simulink model "Sistema_Complejo"  (R2017b)
settings: Solver=FixedStepAuto  StartTime=0.0  StopTime=10.0  FixedStep=0.001  RelTol=1e-3
values from neighbouring files (symbols this model uses):
  B = 20    [Sistema_Complejo.m]    (also in Sistema_Sencillo.m)
  F = 100    [Sistema_Complejo.m]    (also in Sistema_Sencillo.m)
  K1 = 491.1    [Sistema_Complejo.m]
  K2 = 50    [Sistema_Complejo.m]
  K3 = 400    [Sistema_Complejo.m]
  M1 = 5.23    [Sistema_Complejo.m]
  M2 = 2.615    [Sistema_Complejo.m]
  ST = 1    [Sistema_Complejo.m]    (also in Sistema_Sencillo.m)
  VI = 0    [Sistema_Complejo.m]    (also in Sistema_Sencillo.m)
settings Model: Creator=DELL  LastModifiedBy=Wilmer
settings SFSimCC: SimUseLocalCustomCode=on
settings RTWCC: RTWUseLocalCustomCode=on
settings CodeAppCC: StateflowObjectComments=on

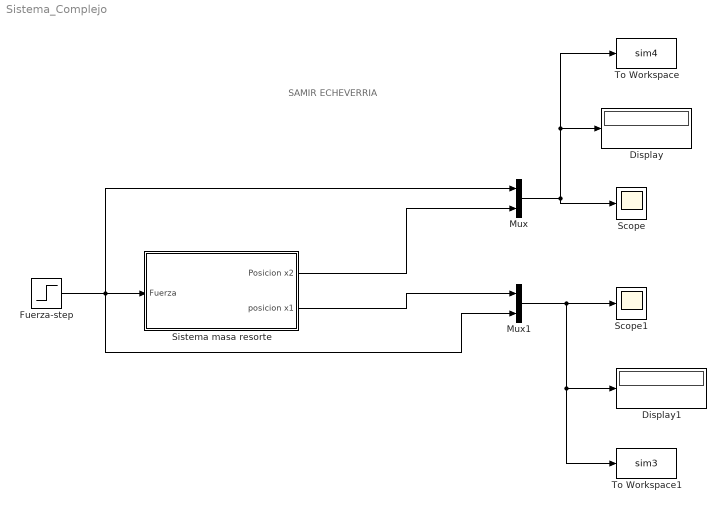
== system Sistema_Complejo ==
  note: SAMIR ECHEVERRIA
  Display : Display
  Display1 : Display
  Fuerza-step : Step  Time=ST  Before=VI  After=F  SampleTime=0
  Mux : Mux  Inputs=2
  Mux1 : Mux  Inputs=2
  Scope : Scope
  Scope1 : Scope
  Sistema masa resorte : Subsystem
  To Workspace : ToWorkspace  VariableName=sim4  SampleTime=-1
  To Workspace1 : ToWorkspace  VariableName=sim3  SampleTime=-1
  wires:
  Fuerza-step/1 -> Mux1/2, Mux/1, Sistema masa resorte/1(Fuerza)
  Sistema masa resorte/1(Posicion x2) -> Mux/2
  Mux/1 -> To Workspace/1, Display/1, Scope/1
  Sistema masa resorte/2("posicion x1 ") -> Mux1/1
  Mux1/1 -> To Workspace1/1, Display1/1, Scope1/1

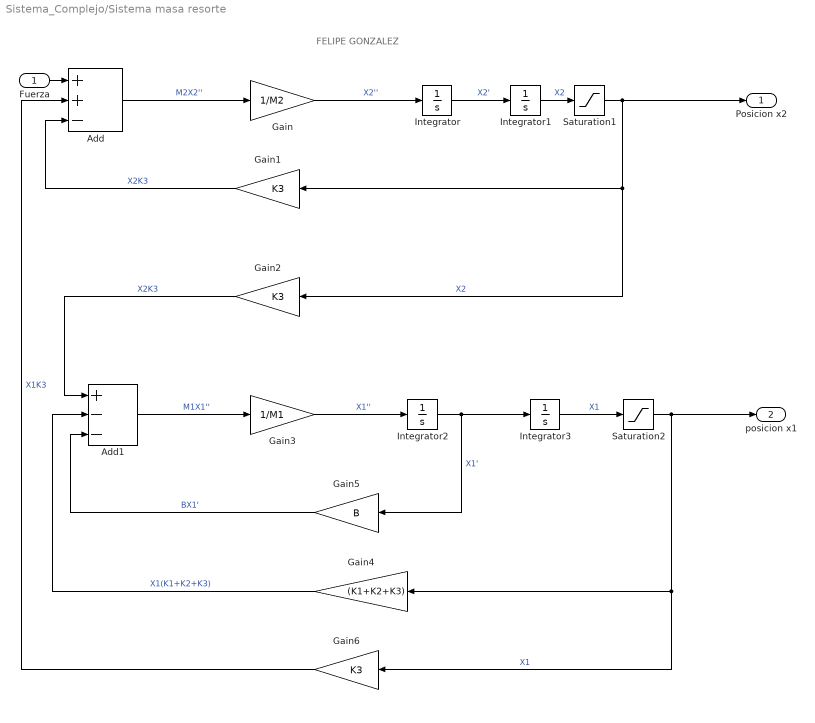
== system Sistema_Complejo/Sistema masa resorte ==
  note: FELIPE GONZALEZ
  Fuerza : Inport
  Add : Sum  Inputs=++-
  Add1 : Sum  Inputs=+--
  Gain : Gain  Gain=1/M2
  Gain1 : Gain  Gain=K3
  Gain2 : Gain  Gain=K3
  Gain3 : Gain  Gain=1/M1
  Gain4 : Gain  Gain=(K1+K2+K3)
  Gain5 : Gain  Gain=B
  Gain6 : Gain  Gain=K3
  Integrator{,1..3} (4 alike) : Integrator
  Saturation1 : Saturate  UpperLimit=0.6  LowerLimit=0
  Saturation2 : Saturate  UpperLimit=1  LowerLimit=0
  Posicion x2 : Outport
  "posicion x1 " : Outport  Port=2
  wires:
  Integrator1/1 -> Saturation1/1  "X2"
  Gain4/1 -> Add1/2  "X1(K1+K2+K3)"
  Integrator3/1 -> Saturation2/1  "X1"
  Integrator2/1 -> Gain5/1, Integrator3/1  "X1'"
  Integrator/1 -> Integrator1/1  "X2'"
  Add/1 -> Gain/1  "M2X2''"
  Gain3/1 -> Integrator2/1  "X1''"
  Add1/1 -> Gain3/1  "M1X1''"
  Gain/1 -> Integrator/1  "X2''"
  Fuerza/1 -> Add/1
  Gain1/1 -> Add/3  "X2K3"
  Gain6/1 -> Add/2  "X1K3"
  Gain5/1 -> Add1/3  "BX1'"
  Gain2/1 -> Add1/1  "X2K3"
  Saturation2/1 -> Gain4/1, Gain6/1, "posicion x1 "/1  "X1"
  Saturation1/1 -> Posicion x2/1, Gain1/1, Gain2/1  "X2"
